simulink model "satellite_sim"  (R2016a)
settings: Solver=ode45  StartTime=0.0  StopTime=200  RelTol=1e-3
InitFcn:
  | param
undefined symbols (not defined in the file or in its folder): drawSatellite, P, satellite_ctrl
settings Model: Creator=beard  LastModifiedBy=beard
settings DataIOCC: LimitDataPoints=on  SaveFormat=Array  SignalLoggingSaveFormat=ModelDataLogs
settings OptimizationCC: ExpressionDepthLimit=2147483647  InitFltsAndDblsToZero=on
settings DebuggingCC: UnderspecifiedInitializationDetection=Classic  MergeDetectMultiDrivingBlocksExec=none  SolverPrmCheckMsg=warning  FcnCallInpInsideContextMsg=UseLocalSettings  StateNameClashWarn=warning
settings HardwareCC: ProdBitPerPointer=32  ProdLargestAtomicFloat=None  ProdIntDivRoundTo=Undefined  ProdEndianess=Unspecified  ProdWordSize=32  ProdHWDeviceType=32-bit Generic
settings ModelReferenceCC: PropagateSignalLabelsOutOfModel=off
settings GRTTargetCC: CombineOutputUpdateFcns=off  GRTInterface=on
settings ConfigComp: CovModelRefEnable=Off

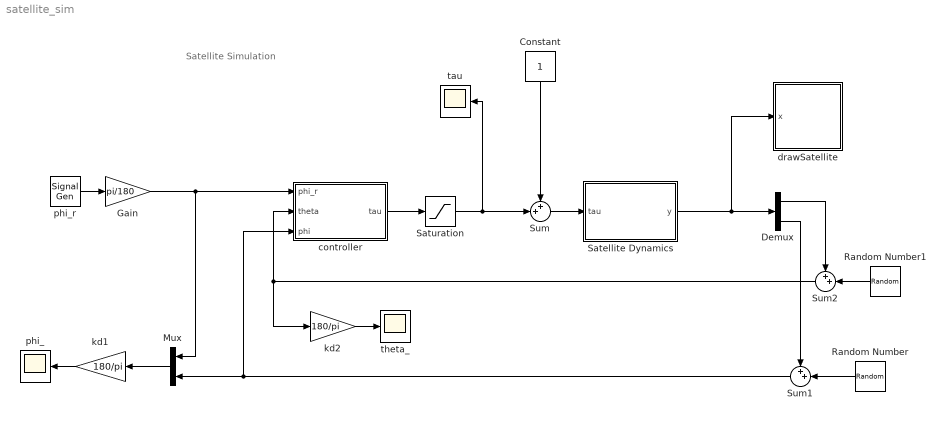
== system satellite_sim ==
  note: Satellite Simulation
  Constant : Constant
  Demux : Demux  Outputs=2
  Gain : Gain  Gain=pi/180
  Mux : Mux  Inputs=2
  Random Number : RandomNumber  Variance=.001^2  SampleTime=0.1
  Random Number1 : RandomNumber  Variance=.001^2  SampleTime=0.1
  Satellite Dynamics : Subsystem
  Saturation : Saturate  UpperLimit=P.taumax  LowerLimit=-P.taumax
  Sum : Sum  Inputs=++|
  Sum1 : Sum  Inputs=++|
  Sum2 : Sum  Inputs=++|
  controller : Subsystem
  drawSatellite : Subsystem
      mask init:
      | % drawing parameters
      | L = 1;
      | w = .3;
      mask Display: image(imread('tv.jpg'))
  kd1 : Gain  Gain=180/pi
  kd2 : Gain  Gain=180/pi
  phi_ : Scope
  phi_r : SignalGenerator  WaveForm=square  Amplitude=15  Frequency=.01
  tau : Scope
  theta_ : Scope
  wires:
  phi_r/1 -> Gain/1
  controller/1(tau) -> Saturation/1
  Gain/1 -> Mux/1, controller/1("phi_r  ")
  kd2/1 -> theta_/1
  Mux/1 -> kd1/1
  kd1/1 -> phi_/1
  Saturation/1 -> tau/1, Sum/2
  Satellite Dynamics/1(y) -> drawSatellite/1(x), Demux/1
  Sum/1 -> Satellite Dynamics/1(tau)
  Demux/1 -> Sum2/1
  Demux/2 -> Sum1/1
  Sum1/1 -> controller/3(phi), Mux/2
  Sum2/1 -> kd2/1, controller/2(theta)
  Random Number1/1 -> Sum2/2
  Random Number/1 -> Sum1/2
  Constant/1 -> Sum/1

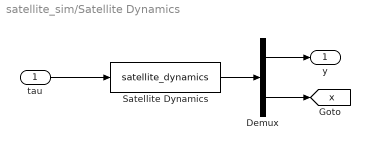
== system satellite_sim/Satellite Dynamics ==
  tau : Inport
  Demux : Demux  Outputs=[2;4]
  Satellite Dynamics : S-Function  FunctionName=satellite_dynamics  Parameters=P  SFunctionDeploymentMode=off  EnableBusSupport=off
  y : Outport
  tag scope: x=global
  wires:
  tau/1 -> Satellite Dynamics/1
  Demux/1 -> y/1
  Satellite Dynamics/1 -> Demux/1
  Demux/2 -> [x]

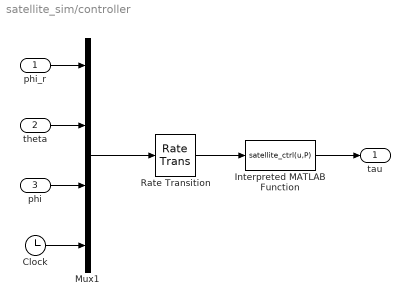
== system satellite_sim/controller ==
  "phi_r  " : Inport
  theta : Inport  Port=2
  phi : Inport  Port=3
  Clock : Clock
  Interpreted MATLAB Function : MATLABFcn  MATLABFcn=satellite_ctrl(u,P)  OutputDimensions=1
  Mux1 : Mux
  Rate Transition : RateTransition  OutPortSampleTime=P.Ts
  tau : Outport
  wires:
  Mux1/1 -> Rate Transition/1
  "phi_r  "/1 -> Mux1/1
  Clock/1 -> Mux1/4
  Rate Transition/1 -> Interpreted MATLAB Function/1
  phi/1 -> Mux1/3
  theta/1 -> Mux1/2
  Interpreted MATLAB Function/1 -> tau/1

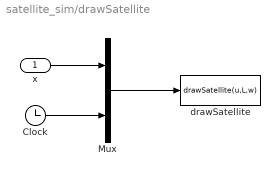
== system satellite_sim/drawSatellite ==
  x : Inport
  Clock : Clock
  Mux : Mux  Inputs=2
  drawSatellite : MATLABFcn  MATLABFcn=drawSatellite(u,L,w)  OutputDimensions=0  SampleTime=0.1
  wires:
  Clock/1 -> Mux/2
  x/1 -> Mux/1
  Mux/1 -> drawSatellite/1
